simulink model "general_charger_2_with_new_rms"  (R2013a)
settings: Solver=ode45  StartTime=0  StopTime=2.5  RelTol=1e-3
PreLoadFcn:
  | Ts =5e-6;
values from neighbouring files (symbols this model uses):
  ac_volt = 169    [charger_init.m]    (also in charger_init_simpl.m)
  Cdc = 2e-3    (= 0.002)    [charger_init.m]    (also in charger_init_simpl.m)
  Lin = 1.5e-3    (= 0.0015)    [charger_init.m]    (also in charger_init_simpl.m = 0.001)
  P = 1.92e3    (= 1920)    [charger_init.m]    (also in charger_init_simpl.m)
  Q = 0    [charger_init.m]    (also in charger_init_simpl.m)
  ramp = (dc_volt - Vdcmin)/(acdc_ramp_end_time)    (= 202)    [charger_init.m]    (also in charger_init_simpl.m = (dc_volt - Vdcmin)/(acdc_ramp_end_time))
  switch_Ts = 5e-5    (= 5e-05)    [charger_init.m]    (also in charger_init_simpl.m)
  sys_Ts = 5e-6    (= 5e-06)    [charger_init.m]    (also in charger_init_simpl.m)
  Vdcmin = ac_volt + 10    (= 179)    [charger_init.m]    (also in charger_init_simpl.m)
  voc = 105    [charger_init.m]    (also in charger_init_simpl.m)
undefined symbols (not defined in the file or in its folder): CESR, DiscIntNeverNeededParam, Rin
undefined symbols (not defined in the file): active_power_on, Ad, Bd, Cd, dc_volt, dcdc_iki, dcdc_ikp, dcdc_on, dcdc_vki, dcdc_vkp, Dd, dq_id_ki, dq_id_kp, dq_iq_ki, dq_iq_kp, dq_vdc_ki, dq_vdc_kp, P_ki, P_kp, Q_ki, Q_kp, reactive_power_on
libraries: simulink_extras x132, powerlib x52, simulink x29, powerlib_meascontrol x8
(part 4 of 5)

== system general_charger_2_with_new_rms/Measurements/Power and angle calculations/discrete low pass filter1/Ad(1,3)/q rounder16 ==
  in : Inport
  Gain9 : Gain  Gain=2^-q
  Idealized ADC quantizer : simulink_extras/Additional Discrete/Idealized ADC quantizer  NumberOfConverterBits=32  Vmin=-range  Vmax=range  OutputDataType=double  OutputNegativeValues=on
  out : Outport
  wires:
  in/1 -> Idealized ADC quantizer/1
  Idealized ADC quantizer/1 -> Gain9/1
  Gain9/1 -> out/1

== system general_charger_2_with_new_rms/Measurements/Power and angle calculations/discrete low pass filter1/Ad(2,1)/q rounder16 ==
  in : Inport
  Gain9 : Gain  Gain=2^-q
  Idealized ADC quantizer : simulink_extras/Additional Discrete/Idealized ADC quantizer  NumberOfConverterBits=32  Vmin=-range  Vmax=range  OutputDataType=double  OutputNegativeValues=on
  out : Outport
  wires:
  in/1 -> Idealized ADC quantizer/1
  Idealized ADC quantizer/1 -> Gain9/1
  Gain9/1 -> out/1

== system general_charger_2_with_new_rms/Measurements/Power and angle calculations/discrete low pass filter1/Ad(2,2)/q rounder16 ==
  in : Inport
  Gain9 : Gain  Gain=2^-q
  Idealized ADC quantizer : simulink_extras/Additional Discrete/Idealized ADC quantizer  NumberOfConverterBits=32  Vmin=-range  Vmax=range  OutputDataType=double  OutputNegativeValues=on
  out : Outport
  wires:
  in/1 -> Idealized ADC quantizer/1
  Idealized ADC quantizer/1 -> Gain9/1
  Gain9/1 -> out/1

== system general_charger_2_with_new_rms/Measurements/Power and angle calculations/discrete low pass filter1/Ad(2,3)/q rounder16 ==
  in : Inport
  Gain9 : Gain  Gain=2^-q
  Idealized ADC quantizer : simulink_extras/Additional Discrete/Idealized ADC quantizer  NumberOfConverterBits=32  Vmin=-range  Vmax=range  OutputDataType=double  OutputNegativeValues=on
  out : Outport
  wires:
  in/1 -> Idealized ADC quantizer/1
  Idealized ADC quantizer/1 -> Gain9/1
  Gain9/1 -> out/1

== system general_charger_2_with_new_rms/Measurements/Power and angle calculations/discrete low pass filter1/Ad(3,1)/q rounder16 ==
  in : Inport
  Gain9 : Gain  Gain=2^-q
  Idealized ADC quantizer : simulink_extras/Additional Discrete/Idealized ADC quantizer  NumberOfConverterBits=32  Vmin=-range  Vmax=range  OutputDataType=double  OutputNegativeValues=on
  out : Outport
  wires:
  in/1 -> Idealized ADC quantizer/1
  Idealized ADC quantizer/1 -> Gain9/1
  Gain9/1 -> out/1

== system general_charger_2_with_new_rms/Measurements/Power and angle calculations/discrete low pass filter1/Ad(3,2)/q rounder16 ==
  in : Inport
  Gain9 : Gain  Gain=2^-q
  Idealized ADC quantizer : simulink_extras/Additional Discrete/Idealized ADC quantizer  NumberOfConverterBits=32  Vmin=-range  Vmax=range  OutputDataType=double  OutputNegativeValues=on
  out : Outport
  wires:
  in/1 -> Idealized ADC quantizer/1
  Idealized ADC quantizer/1 -> Gain9/1
  Gain9/1 -> out/1

== system general_charger_2_with_new_rms/Measurements/Power and angle calculations/discrete low pass filter1/Ad(3,3)/q rounder16 ==
  in : Inport
  Gain9 : Gain  Gain=2^-q
  Idealized ADC quantizer : simulink_extras/Additional Discrete/Idealized ADC quantizer  NumberOfConverterBits=32  Vmin=-range  Vmax=range  OutputDataType=double  OutputNegativeValues=on
  out : Outport
  wires:
  in/1 -> Idealized ADC quantizer/1
  Idealized ADC quantizer/1 -> Gain9/1
  Gain9/1 -> out/1

== system general_charger_2_with_new_rms/Measurements/Power and angle calculations/discrete low pass filter1/Bd(1)/q rounder16 ==
  in : Inport
  Gain9 : Gain  Gain=2^-q
  Idealized ADC quantizer : simulink_extras/Additional Discrete/Idealized ADC quantizer  NumberOfConverterBits=32  Vmin=-range  Vmax=range  OutputDataType=double  OutputNegativeValues=on
  out : Outport
  wires:
  in/1 -> Idealized ADC quantizer/1
  Idealized ADC quantizer/1 -> Gain9/1
  Gain9/1 -> out/1

== system general_charger_2_with_new_rms/Measurements/Power and angle calculations/discrete low pass filter1/Bd(2)/q rounder16 ==
  in : Inport
  Gain9 : Gain  Gain=2^-q
  Idealized ADC quantizer : simulink_extras/Additional Discrete/Idealized ADC quantizer  NumberOfConverterBits=32  Vmin=-range  Vmax=range  OutputDataType=double  OutputNegativeValues=on
  out : Outport
  wires:
  in/1 -> Idealized ADC quantizer/1
  Idealized ADC quantizer/1 -> Gain9/1
  Gain9/1 -> out/1

== system general_charger_2_with_new_rms/Measurements/Power and angle calculations/discrete low pass filter1/Bd(3)/q rounder16 ==
  in : Inport
  Gain9 : Gain  Gain=2^-q
  Idealized ADC quantizer : simulink_extras/Additional Discrete/Idealized ADC quantizer  NumberOfConverterBits=32  Vmin=-range  Vmax=range  OutputDataType=double  OutputNegativeValues=on
  out : Outport
  wires:
  in/1 -> Idealized ADC quantizer/1
  Idealized ADC quantizer/1 -> Gain9/1
  Gain9/1 -> out/1

== system general_charger_2_with_new_rms/Measurements/Power and angle calculations/discrete low pass filter1/Cd(1)/q rounder16 ==
  in : Inport
  Gain9 : Gain  Gain=2^-q
  Idealized ADC quantizer : simulink_extras/Additional Discrete/Idealized ADC quantizer  NumberOfConverterBits=32  Vmin=-range  Vmax=range  OutputDataType=double  OutputNegativeValues=on
  out : Outport
  wires:
  in/1 -> Idealized ADC quantizer/1
  Idealized ADC quantizer/1 -> Gain9/1
  Gain9/1 -> out/1

== system general_charger_2_with_new_rms/Measurements/Power and angle calculations/discrete low pass filter1/Cd(2)/q rounder16 ==
  in : Inport
  Gain9 : Gain  Gain=2^-q
  Idealized ADC quantizer : simulink_extras/Additional Discrete/Idealized ADC quantizer  NumberOfConverterBits=32  Vmin=-range  Vmax=range  OutputDataType=double  OutputNegativeValues=on
  out : Outport
  wires:
  in/1 -> Idealized ADC quantizer/1
  Idealized ADC quantizer/1 -> Gain9/1
  Gain9/1 -> out/1

== system general_charger_2_with_new_rms/Measurements/Power and angle calculations/discrete low pass filter1/Cd(3)/q rounder16 ==
  in : Inport
  Gain9 : Gain  Gain=2^-q
  Idealized ADC quantizer : simulink_extras/Additional Discrete/Idealized ADC quantizer  NumberOfConverterBits=32  Vmin=-range  Vmax=range  OutputDataType=double  OutputNegativeValues=on
  out : Outport
  wires:
  in/1 -> Idealized ADC quantizer/1
  Idealized ADC quantizer/1 -> Gain9/1
  Gain9/1 -> out/1

== system general_charger_2_with_new_rms/Measurements/Power and angle calculations/discrete low pass filter1/Dd/q rounder16 ==
  in : Inport
  Gain9 : Gain  Gain=2^-q
  Idealized ADC quantizer : simulink_extras/Additional Discrete/Idealized ADC quantizer  NumberOfConverterBits=32  Vmin=-range  Vmax=range  OutputDataType=double  OutputNegativeValues=on
  out : Outport
  wires:
  in/1 -> Idealized ADC quantizer/1
  Idealized ADC quantizer/1 -> Gain9/1
  Gain9/1 -> out/1

== system general_charger_2_with_new_rms/Measurements/Power and angle calculations/discrete low pass filter2/Ad(1,1)/q rounder16 ==
  in : Inport
  Gain9 : Gain  Gain=2^-q
  Idealized ADC quantizer : simulink_extras/Additional Discrete/Idealized ADC quantizer  NumberOfConverterBits=32  Vmin=-range  Vmax=range  OutputDataType=double  OutputNegativeValues=on
  out : Outport
  wires:
  in/1 -> Idealized ADC quantizer/1
  Idealized ADC quantizer/1 -> Gain9/1
  Gain9/1 -> out/1

== system general_charger_2_with_new_rms/Measurements/Power and angle calculations/discrete low pass filter2/Ad(1,2)/q rounder16 ==
  in : Inport
  Gain9 : Gain  Gain=2^-q
  Idealized ADC quantizer : simulink_extras/Additional Discrete/Idealized ADC quantizer  NumberOfConverterBits=32  Vmin=-range  Vmax=range  OutputDataType=double  OutputNegativeValues=on
  out : Outport
  wires:
  in/1 -> Idealized ADC quantizer/1
  Idealized ADC quantizer/1 -> Gain9/1
  Gain9/1 -> out/1

== system general_charger_2_with_new_rms/Measurements/Power and angle calculations/discrete low pass filter2/Ad(1,3)/q rounder16 ==
  in : Inport
  Gain9 : Gain  Gain=2^-q
  Idealized ADC quantizer : simulink_extras/Additional Discrete/Idealized ADC quantizer  NumberOfConverterBits=32  Vmin=-range  Vmax=range  OutputDataType=double  OutputNegativeValues=on
  out : Outport
  wires:
  in/1 -> Idealized ADC quantizer/1
  Idealized ADC quantizer/1 -> Gain9/1
  Gain9/1 -> out/1

== system general_charger_2_with_new_rms/Measurements/Power and angle calculations/discrete low pass filter2/Ad(2,1)/q rounder16 ==
  in : Inport
  Gain9 : Gain  Gain=2^-q
  Idealized ADC quantizer : simulink_extras/Additional Discrete/Idealized ADC quantizer  NumberOfConverterBits=32  Vmin=-range  Vmax=range  OutputDataType=double  OutputNegativeValues=on
  out : Outport
  wires:
  in/1 -> Idealized ADC quantizer/1
  Idealized ADC quantizer/1 -> Gain9/1
  Gain9/1 -> out/1

== system general_charger_2_with_new_rms/Measurements/Power and angle calculations/discrete low pass filter2/Ad(2,2)/q rounder16 ==
  in : Inport
  Gain9 : Gain  Gain=2^-q
  Idealized ADC quantizer : simulink_extras/Additional Discrete/Idealized ADC quantizer  NumberOfConverterBits=32  Vmin=-range  Vmax=range  OutputDataType=double  OutputNegativeValues=on
  out : Outport
  wires:
  in/1 -> Idealized ADC quantizer/1
  Idealized ADC quantizer/1 -> Gain9/1
  Gain9/1 -> out/1

== system general_charger_2_with_new_rms/Measurements/Power and angle calculations/discrete low pass filter2/Ad(2,3)/q rounder16 ==
  in : Inport
  Gain9 : Gain  Gain=2^-q
  Idealized ADC quantizer : simulink_extras/Additional Discrete/Idealized ADC quantizer  NumberOfConverterBits=32  Vmin=-range  Vmax=range  OutputDataType=double  OutputNegativeValues=on
  out : Outport
  wires:
  in/1 -> Idealized ADC quantizer/1
  Idealized ADC quantizer/1 -> Gain9/1
  Gain9/1 -> out/1

== system general_charger_2_with_new_rms/Measurements/Power and angle calculations/discrete low pass filter2/Ad(3,1)/q rounder16 ==
  in : Inport
  Gain9 : Gain  Gain=2^-q
  Idealized ADC quantizer : simulink_extras/Additional Discrete/Idealized ADC quantizer  NumberOfConverterBits=32  Vmin=-range  Vmax=range  OutputDataType=double  OutputNegativeValues=on
  out : Outport
  wires:
  in/1 -> Idealized ADC quantizer/1
  Idealized ADC quantizer/1 -> Gain9/1
  Gain9/1 -> out/1

== system general_charger_2_with_new_rms/Measurements/Power and angle calculations/discrete low pass filter2/Ad(3,2)/q rounder16 ==
  in : Inport
  Gain9 : Gain  Gain=2^-q
  Idealized ADC quantizer : simulink_extras/Additional Discrete/Idealized ADC quantizer  NumberOfConverterBits=32  Vmin=-range  Vmax=range  OutputDataType=double  OutputNegativeValues=on
  out : Outport
  wires:
  in/1 -> Idealized ADC quantizer/1
  Idealized ADC quantizer/1 -> Gain9/1
  Gain9/1 -> out/1

== system general_charger_2_with_new_rms/Measurements/Power and angle calculations/discrete low pass filter2/Ad(3,3)/q rounder16 ==
  in : Inport
  Gain9 : Gain  Gain=2^-q
  Idealized ADC quantizer : simulink_extras/Additional Discrete/Idealized ADC quantizer  NumberOfConverterBits=32  Vmin=-range  Vmax=range  OutputDataType=double  OutputNegativeValues=on
  out : Outport
  wires:
  in/1 -> Idealized ADC quantizer/1
  Idealized ADC quantizer/1 -> Gain9/1
  Gain9/1 -> out/1

== system general_charger_2_with_new_rms/Measurements/Power and angle calculations/discrete low pass filter2/Bd(1)/q rounder16 ==
  in : Inport
  Gain9 : Gain  Gain=2^-q
  Idealized ADC quantizer : simulink_extras/Additional Discrete/Idealized ADC quantizer  NumberOfConverterBits=32  Vmin=-range  Vmax=range  OutputDataType=double  OutputNegativeValues=on
  out : Outport
  wires:
  in/1 -> Idealized ADC quantizer/1
  Idealized ADC quantizer/1 -> Gain9/1
  Gain9/1 -> out/1

== system general_charger_2_with_new_rms/Measurements/Power and angle calculations/discrete low pass filter2/Bd(2)/q rounder16 ==
  in : Inport
  Gain9 : Gain  Gain=2^-q
  Idealized ADC quantizer : simulink_extras/Additional Discrete/Idealized ADC quantizer  NumberOfConverterBits=32  Vmin=-range  Vmax=range  OutputDataType=double  OutputNegativeValues=on
  out : Outport
  wires:
  in/1 -> Idealized ADC quantizer/1
  Idealized ADC quantizer/1 -> Gain9/1
  Gain9/1 -> out/1

== system general_charger_2_with_new_rms/Measurements/Power and angle calculations/discrete low pass filter2/Bd(3)/q rounder16 ==
  in : Inport
  Gain9 : Gain  Gain=2^-q
  Idealized ADC quantizer : simulink_extras/Additional Discrete/Idealized ADC quantizer  NumberOfConverterBits=32  Vmin=-range  Vmax=range  OutputDataType=double  OutputNegativeValues=on
  out : Outport
  wires:
  in/1 -> Idealized ADC quantizer/1
  Idealized ADC quantizer/1 -> Gain9/1
  Gain9/1 -> out/1

== system general_charger_2_with_new_rms/Measurements/Power and angle calculations/discrete low pass filter2/Cd(1)/q rounder16 ==
  in : Inport
  Gain9 : Gain  Gain=2^-q
  Idealized ADC quantizer : simulink_extras/Additional Discrete/Idealized ADC quantizer  NumberOfConverterBits=32  Vmin=-range  Vmax=range  OutputDataType=double  OutputNegativeValues=on
  out : Outport
  wires:
  in/1 -> Idealized ADC quantizer/1
  Idealized ADC quantizer/1 -> Gain9/1
  Gain9/1 -> out/1

== system general_charger_2_with_new_rms/Measurements/Power and angle calculations/discrete low pass filter2/Cd(2)/q rounder16 ==
  in : Inport
  Gain9 : Gain  Gain=2^-q
  Idealized ADC quantizer : simulink_extras/Additional Discrete/Idealized ADC quantizer  NumberOfConverterBits=32  Vmin=-range  Vmax=range  OutputDataType=double  OutputNegativeValues=on
  out : Outport
  wires:
  in/1 -> Idealized ADC quantizer/1
  Idealized ADC quantizer/1 -> Gain9/1
  Gain9/1 -> out/1

== system general_charger_2_with_new_rms/Measurements/Power and angle calculations/discrete low pass filter2/Cd(3)/q rounder16 ==
  in : Inport
  Gain9 : Gain  Gain=2^-q
  Idealized ADC quantizer : simulink_extras/Additional Discrete/Idealized ADC quantizer  NumberOfConverterBits=32  Vmin=-range  Vmax=range  OutputDataType=double  OutputNegativeValues=on
  out : Outport
  wires:
  in/1 -> Idealized ADC quantizer/1
  Idealized ADC quantizer/1 -> Gain9/1
  Gain9/1 -> out/1

== system general_charger_2_with_new_rms/Measurements/Power and angle calculations/discrete low pass filter2/Dd/q rounder16 ==
  in : Inport
  Gain9 : Gain  Gain=2^-q
  Idealized ADC quantizer : simulink_extras/Additional Discrete/Idealized ADC quantizer  NumberOfConverterBits=32  Vmin=-range  Vmax=range  OutputDataType=double  OutputNegativeValues=on
  out : Outport
  wires:
  in/1 -> Idealized ADC quantizer/1
  Idealized ADC quantizer/1 -> Gain9/1
  Gain9/1 -> out/1

== system general_charger_2_with_new_rms/Measurements/THD/discrete low pass filter1/Ad(1,1)/q rounder16 ==
  in : Inport
  Gain9 : Gain  Gain=2^-q
  Idealized ADC quantizer : simulink_extras/Additional Discrete/Idealized ADC quantizer  NumberOfConverterBits=32  Vmin=-range  Vmax=range  OutputDataType=double  OutputNegativeValues=on
  out : Outport
  wires:
  in/1 -> Idealized ADC quantizer/1
  Idealized ADC quantizer/1 -> Gain9/1
  Gain9/1 -> out/1

== system general_charger_2_with_new_rms/Measurements/THD/discrete low pass filter1/Ad(1,2)/q rounder16 ==
  in : Inport
  Gain9 : Gain  Gain=2^-q
  Idealized ADC quantizer : simulink_extras/Additional Discrete/Idealized ADC quantizer  NumberOfConverterBits=32  Vmin=-range  Vmax=range  OutputDataType=double  OutputNegativeValues=on
  out : Outport
  wires:
  in/1 -> Idealized ADC quantizer/1
  Idealized ADC quantizer/1 -> Gain9/1
  Gain9/1 -> out/1

== system general_charger_2_with_new_rms/Measurements/THD/discrete low pass filter1/Ad(1,3)/q rounder16 ==
  in : Inport
  Gain9 : Gain  Gain=2^-q
  Idealized ADC quantizer : simulink_extras/Additional Discrete/Idealized ADC quantizer  NumberOfConverterBits=32  Vmin=-range  Vmax=range  OutputDataType=double  OutputNegativeValues=on
  out : Outport
  wires:
  in/1 -> Idealized ADC quantizer/1
  Idealized ADC quantizer/1 -> Gain9/1
  Gain9/1 -> out/1

== system general_charger_2_with_new_rms/Measurements/THD/discrete low pass filter1/Ad(2,1)/q rounder16 ==
  in : Inport
  Gain9 : Gain  Gain=2^-q
  Idealized ADC quantizer : simulink_extras/Additional Discrete/Idealized ADC quantizer  NumberOfConverterBits=32  Vmin=-range  Vmax=range  OutputDataType=double  OutputNegativeValues=on
  out : Outport
  wires:
  in/1 -> Idealized ADC quantizer/1
  Idealized ADC quantizer/1 -> Gain9/1
  Gain9/1 -> out/1

== system general_charger_2_with_new_rms/Measurements/THD/discrete low pass filter1/Ad(2,2)/q rounder16 ==
  in : Inport
  Gain9 : Gain  Gain=2^-q
  Idealized ADC quantizer : simulink_extras/Additional Discrete/Idealized ADC quantizer  NumberOfConverterBits=32  Vmin=-range  Vmax=range  OutputDataType=double  OutputNegativeValues=on
  out : Outport
  wires:
  in/1 -> Idealized ADC quantizer/1
  Idealized ADC quantizer/1 -> Gain9/1
  Gain9/1 -> out/1

== system general_charger_2_with_new_rms/Measurements/THD/discrete low pass filter1/Ad(2,3)/q rounder16 ==
  in : Inport
  Gain9 : Gain  Gain=2^-q
  Idealized ADC quantizer : simulink_extras/Additional Discrete/Idealized ADC quantizer  NumberOfConverterBits=32  Vmin=-range  Vmax=range  OutputDataType=double  OutputNegativeValues=on
  out : Outport
  wires:
  in/1 -> Idealized ADC quantizer/1
  Idealized ADC quantizer/1 -> Gain9/1
  Gain9/1 -> out/1

== system general_charger_2_with_new_rms/Measurements/THD/discrete low pass filter1/Ad(3,1)/q rounder16 ==
  in : Inport
  Gain9 : Gain  Gain=2^-q
  Idealized ADC quantizer : simulink_extras/Additional Discrete/Idealized ADC quantizer  NumberOfConverterBits=32  Vmin=-range  Vmax=range  OutputDataType=double  OutputNegativeValues=on
  out : Outport
  wires:
  in/1 -> Idealized ADC quantizer/1
  Idealized ADC quantizer/1 -> Gain9/1
  Gain9/1 -> out/1

== system general_charger_2_with_new_rms/Measurements/THD/discrete low pass filter1/Ad(3,2)/q rounder16 ==
  in : Inport
  Gain9 : Gain  Gain=2^-q
  Idealized ADC quantizer : simulink_extras/Additional Discrete/Idealized ADC quantizer  NumberOfConverterBits=32  Vmin=-range  Vmax=range  OutputDataType=double  OutputNegativeValues=on
  out : Outport
  wires:
  in/1 -> Idealized ADC quantizer/1
  Idealized ADC quantizer/1 -> Gain9/1
  Gain9/1 -> out/1

== system general_charger_2_with_new_rms/Measurements/THD/discrete low pass filter1/Ad(3,3)/q rounder16 ==
  in : Inport
  Gain9 : Gain  Gain=2^-q
  Idealized ADC quantizer : simulink_extras/Additional Discrete/Idealized ADC quantizer  NumberOfConverterBits=32  Vmin=-range  Vmax=range  OutputDataType=double  OutputNegativeValues=on
  out : Outport
  wires:
  in/1 -> Idealized ADC quantizer/1
  Idealized ADC quantizer/1 -> Gain9/1
  Gain9/1 -> out/1

== system general_charger_2_with_new_rms/Measurements/THD/discrete low pass filter1/Bd(1)/q rounder16 ==
  in : Inport
  Gain9 : Gain  Gain=2^-q
  Idealized ADC quantizer : simulink_extras/Additional Discrete/Idealized ADC quantizer  NumberOfConverterBits=32  Vmin=-range  Vmax=range  OutputDataType=double  OutputNegativeValues=on
  out : Outport
  wires:
  in/1 -> Idealized ADC quantizer/1
  Idealized ADC quantizer/1 -> Gain9/1
  Gain9/1 -> out/1

== system general_charger_2_with_new_rms/Measurements/THD/discrete low pass filter1/Bd(2)/q rounder16 ==
  in : Inport
  Gain9 : Gain  Gain=2^-q
  Idealized ADC quantizer : simulink_extras/Additional Discrete/Idealized ADC quantizer  NumberOfConverterBits=32  Vmin=-range  Vmax=range  OutputDataType=double  OutputNegativeValues=on
  out : Outport
  wires:
  in/1 -> Idealized ADC quantizer/1
  Idealized ADC quantizer/1 -> Gain9/1
  Gain9/1 -> out/1

== system general_charger_2_with_new_rms/Measurements/THD/discrete low pass filter1/Bd(3)/q rounder16 ==
  in : Inport
  Gain9 : Gain  Gain=2^-q
  Idealized ADC quantizer : simulink_extras/Additional Discrete/Idealized ADC quantizer  NumberOfConverterBits=32  Vmin=-range  Vmax=range  OutputDataType=double  OutputNegativeValues=on
  out : Outport
  wires:
  in/1 -> Idealized ADC quantizer/1
  Idealized ADC quantizer/1 -> Gain9/1
  Gain9/1 -> out/1

== system general_charger_2_with_new_rms/Measurements/THD/discrete low pass filter1/Cd(1)/q rounder16 ==
  in : Inport
  Gain9 : Gain  Gain=2^-q
  Idealized ADC quantizer : simulink_extras/Additional Discrete/Idealized ADC quantizer  NumberOfConverterBits=32  Vmin=-range  Vmax=range  OutputDataType=double  OutputNegativeValues=on
  out : Outport
  wires:
  in/1 -> Idealized ADC quantizer/1
  Idealized ADC quantizer/1 -> Gain9/1
  Gain9/1 -> out/1

== system general_charger_2_with_new_rms/Measurements/THD/discrete low pass filter1/Cd(2)/q rounder16 ==
  in : Inport
  Gain9 : Gain  Gain=2^-q
  Idealized ADC quantizer : simulink_extras/Additional Discrete/Idealized ADC quantizer  NumberOfConverterBits=32  Vmin=-range  Vmax=range  OutputDataType=double  OutputNegativeValues=on
  out : Outport
  wires:
  in/1 -> Idealized ADC quantizer/1
  Idealized ADC quantizer/1 -> Gain9/1
  Gain9/1 -> out/1

== system general_charger_2_with_new_rms/Measurements/THD/discrete low pass filter1/Cd(3)/q rounder16 ==
  in : Inport
  Gain9 : Gain  Gain=2^-q
  Idealized ADC quantizer : simulink_extras/Additional Discrete/Idealized ADC quantizer  NumberOfConverterBits=32  Vmin=-range  Vmax=range  OutputDataType=double  OutputNegativeValues=on
  out : Outport
  wires:
  in/1 -> Idealized ADC quantizer/1
  Idealized ADC quantizer/1 -> Gain9/1
  Gain9/1 -> out/1

== system general_charger_2_with_new_rms/Measurements/THD/discrete low pass filter1/Dd/q rounder16 ==
  in : Inport
  Gain9 : Gain  Gain=2^-q
  Idealized ADC quantizer : simulink_extras/Additional Discrete/Idealized ADC quantizer  NumberOfConverterBits=32  Vmin=-range  Vmax=range  OutputDataType=double  OutputNegativeValues=on
  out : Outport
  wires:
  in/1 -> Idealized ADC quantizer/1
  Idealized ADC quantizer/1 -> Gain9/1
  Gain9/1 -> out/1

== system general_charger_2_with_new_rms/control_stage/AC//DC Control/DQ Controller/AB-DQ Transform/AB->DQ ==
  A : Inport
  wt : Inport  Port=2
  phi : Inport  Port=3
  Add1 : Sum  Inputs=-+
  Add2 : Sum
  Delay : Delay  DelayLength=RSpC  SampleTime=abdq_Ts
  Gain : Gain  Gain=-1
  Id Discretization Error Correction : Subsystem
  Iq Discretization Error Correction : Subsystem
  Product{1..4} (4 alike) : Product  RndMeth=Zero
  Trigonometric Function : Trigonometry
  Trigonometric Function1 : Trigonometry  Operator=cos
  Unit Delay : UnitDelay  SampleTime=switch_Ts
  D : Outport
  Q : Outport  Port=2
  wires:
  Trigonometric Function/1 -> Product1/1, Product2/1
  Product1/1 -> Add2/2
  Product4/1 -> Add2/1
  Product2/1 -> Add1/1
  A/1 -> Iq Discretization Error Correction/4(A), Delay/1, Id Discretization Error Correction/1(A), Product4/1, Product2/2
  Trigonometric Function1/1 -> Product4/2, Product3/1
  Product3/1 -> Add1/2
  Delay/1 -> Product1/2, Product3/2  "B"
  wt/1 -> [theta], Trigonometric Function1/1, Trigonometric Function/1
  Add2/1 -> Id Discretization Error Correction/3(D)  "Vd"
  Add1/1 -> Iq Discretization Error Correction/2(Q)
  [theta] -> Iq Discretization Error Correction/3(wt)
  [theta] -> Id Discretization Error Correction/2(wt)
  Id Discretization Error Correction/1(Id_corr) -> D/1
  Iq Discretization Error Correction/1(Iq_corr) -> Q/1
  phi/1 -> Gain/1
  Unit Delay/1 -> Iq Discretization Error Correction/1(phi), Id Discretization Error Correction/4(phi)
  Gain/1 -> Unit Delay/1

== system general_charger_2_with_new_rms/control_stage/AC//DC Control/DQ Controller/AB-DQ Transform/PLL ==
  note: PLL based on dq frame control
      | input signal is assumed to be 60 Hz
      | and sample time is 50e-6
  signal_in : Inport
  AB->DQ : Subsystem  mask{abdq_f=pll_f, abdq_Ts=pll_Ts}
      mask prompts: abdq_f "frequency"; abdq_Ts "Sample Time"
      mask init:
      | SpC=1/abdq_f/4/abdq_Ts;
      | RSpC=ceil(SpC);
  Constant1 : Constant  Value=0
  Constant3 : Constant  Value=2*pi*pll_f
  PI1 : Subsystem  mask{ki=1, kp=0, Ts_pi=pll_Ts, int_sat_up=inf, int_sat_low=-inf, pi_sat_up=inf, pi_sat_low=-inf}
      mask prompts: ki "Integral Gain"; kp "Proportional Gain"; Ts_pi "Sample Time"; int_sat_up "Integral Saturation Upper"; int_sat_low "Integral Saturation Lower"; pi_sat_up "PI Controller Saturation Upper"; pi_sat_low "PI Controller Saturation Lower"
      mask Display: disp('PI')
  PI4 : Subsystem  mask{ki=pll_ki, kp=pll_kp, Ts_pi=pll_Ts, int_sat_up=inf, int_sat_low=-inf, pi_sat_up=inf, pi_sat_low=-inf}
      mask prompts: ki "Integral Gain"; kp "Proportional Gain"; Ts_pi "Sample Time"; int_sat_up "Integral Saturation Upper"; int_sat_low "Integral Saturation Lower"; pi_sat_up "PI Controller Saturation Upper"; pi_sat_low "PI Controller Saturation Lower"
      mask Display: disp('PI')
  Sum : Sum  Inputs=|-+
  Sum2 : Sum  Inputs=|-+
  angle_out : Outport
  D : Outport  Port=2
  Q : Outport  Port=3
  wires:
  Constant1/1 -> Sum/2
  Sum/1 -> PI4/1(in)
  PI1/1(out) -> angle_out/1, AB->DQ/2(wt)
  Constant3/1 -> Sum2/2
  PI4/1(out) -> Sum2/1
  AB->DQ/2(Q) -> Q/1, Sum/1
  signal_in/1 -> AB->DQ/1(A)
  AB->DQ/1(D) -> D/1
  Sum2/1 -> PI1/1(in)  "pll_int_error"

== system general_charger_2_with_new_rms/control_stage/AC//DC Control/DQ Controller/DQ Controller Submodule/DQ-->A ==
  D : Inport
  Q : Inport  Port=2
  wt : Inport  Port=3
  Add2 : Sum  Inputs=+-
  Product1 : Product  RndMeth=Zero
  Product4 : Product  RndMeth=Zero
  Trigonometric Function : Trigonometry
  Trigonometric Function1 : Trigonometry  Operator=cos
  A : Outport
  wires:
  Add2/1 -> A/1  "Vd"
  Product1/1 -> Add2/2
  Product4/1 -> Add2/1
  wt/1 -> Trigonometric Function1/1, Trigonometric Function/1
  Trigonometric Function1/1 -> Product4/2
  D/1 -> Product4/1
  Q/1 -> Product1/2
  Trigonometric Function/1 -> Product1/1

== system general_charger_2_with_new_rms/control_stage/AC//DC Control/DQ Controller/DQ Controller Submodule/PI1 ==
  in : Inport
  Add1 : Sum
  Add2 : Sum
  Ki : Gain  Gain=ki
  Kp : Gain  Gain=kp
  Tappe : simulink/Discrete/Tapped Delay  vinit=0.0  samptime=Ts_pi  NumDelays=1  DelayOrder=Oldest  includeCurrent=off
  Ts : Gain  Gain=Ts_pi
  integral saturation : Saturate  UpperLimit=int_sat_up  LowerLimit=int_sat_low  SampleTime=Ts_pi
  pi controller saturation : Saturate  UpperLimit=pi_sat_up  LowerLimit=pi_sat_low  SampleTime=Ts_pi
  out : Outport
  wires:
  Ts/1 -> Ki/1
  in/1 -> Kp/1, Ts/1  "vdc_error"
  Add1/1 -> integral saturation/1  "vdc_int_pi"
  Kp/1 -> Add2/2  "vdc_kp_pi"
  pi controller saturation/1 -> out/1
  Tappe/1 -> Add1/1
  Add2/1 -> pi controller saturation/1  "vdc_pi"
  Ki/1 -> Add1/2
  integral saturation/1 -> Add2/1, Tappe/1

== system general_charger_2_with_new_rms/control_stage/AC//DC Control/DQ Controller/DQ Controller Submodule/PI2 ==
  in : Inport
  Add1 : Sum
  Add2 : Sum
  Ki : Gain  Gain=ki
  Kp : Gain  Gain=kp
  Tappe : simulink/Discrete/Tapped Delay  vinit=0.0  samptime=Ts_pi  NumDelays=1  DelayOrder=Oldest  includeCurrent=off
  Ts : Gain  Gain=Ts_pi
  integral saturation : Saturate  UpperLimit=int_sat_up  LowerLimit=int_sat_low  SampleTime=Ts_pi
  pi controller saturation : Saturate  UpperLimit=pi_sat_up  LowerLimit=pi_sat_low  SampleTime=Ts_pi
  out : Outport
  wires:
  Ts/1 -> Ki/1
  in/1 -> Kp/1, Ts/1  "vdc_error"
  Add1/1 -> integral saturation/1  "vdc_int_pi"
  Kp/1 -> Add2/2  "vdc_kp_pi"
  pi controller saturation/1 -> out/1
  Tappe/1 -> Add1/1
  Add2/1 -> pi controller saturation/1  "vdc_pi"
  Ki/1 -> Add1/2
  integral saturation/1 -> Add2/1, Tappe/1

== system general_charger_2_with_new_rms/control_stage/AC//DC Control/DQ Controller/DQ Controller Submodule/PI3 ==
  in : Inport
  Add1 : Sum
  Add2 : Sum
  Ki : Gain  Gain=ki
  Kp : Gain  Gain=kp
  Tappe : simulink/Discrete/Tapped Delay  vinit=0.0  samptime=Ts_pi  NumDelays=1  DelayOrder=Oldest  includeCurrent=off
  Ts : Gain  Gain=Ts_pi
  integral saturation : Saturate  UpperLimit=int_sat_up  LowerLimit=int_sat_low  SampleTime=Ts_pi
  pi controller saturation : Saturate  UpperLimit=pi_sat_up  LowerLimit=pi_sat_low  SampleTime=Ts_pi
  out : Outport
  wires:
  Ts/1 -> Ki/1
  in/1 -> Kp/1, Ts/1  "vdc_error"
  Add1/1 -> integral saturation/1  "vdc_int_pi"
  Kp/1 -> Add2/2  "vdc_kp_pi"
  pi controller saturation/1 -> out/1
  Tappe/1 -> Add1/1
  Add2/1 -> pi controller saturation/1  "vdc_pi"
  Ki/1 -> Add1/2
  integral saturation/1 -> Add2/1, Tappe/1

== system general_charger_2_with_new_rms/control_stage/AC//DC Control/DQ Controller/DQ Controller Submodule/Reactive Power Control Module ==
  Add8 : Sum  Inputs=+-
  Constant1 : Constant  Value=Q
  Constant3 : Constant  Value=0
  Divide2 : Product  Inputs=/*  InputSameDT=on
  Gain4 : Gain  Gain=0.5
  Gain5 : Gain  Gain=-1
  PI4 : Subsystem  mask{ki=Q_ki, kp=Q_kp, Ts_pi=Ts, int_sat_up=inf, int_sat_low=-inf, pi_sat_up=inf, pi_sat_low=-inf}
      mask prompts: ki "Integral Gain"; kp "Proportional Gain"; Ts_pi "Sample Time"; int_sat_up "Integral Saturation Upper"; int_sat_low "Integral Saturation Lower"; pi_sat_up "PI Controller Saturation Upper"; pi_sat_low "PI Controller Saturation Lower"
      mask Display: disp('PI')
  Saturation : Saturate  UpperLimit=inf  LowerLimit=1
  Step1 : Step  Time=turn_on  SampleTime=0
  Switch3 : Switch  Threshold=0.5
  Iq_ref : Outport
  wires:
  PI4/1(out) -> Iq_ref/1
  Gain4/1 -> Divide2/1
  Divide2/1 -> PI4/1(in)
  Saturation/1 -> Gain4/1
  Gain5/1 -> Switch3/1
  Constant3/1 -> Switch3/3
  Constant1/1 -> Add8/1
  [Qpower] -> Add8/2
  Step1/1 -> Switch3/2
  [nVd] -> Saturation/1
  Switch3/1 -> Divide2/2
  Add8/1 -> Gain5/1

== system general_charger_2_with_new_rms/control_stage/AC//DC Control/DQ Controller/discrete low pass filter1/Ad(1,1) ==
  in : Inport
  Constant1 : Constant  Value=variable
  Product1 : Product
  q rounder16 : Subsystem  mask{q=nQ, range=maxRange}
      mask prompts: q "q value"; range "q range"
  out : Outport
  wires:
  q rounder16/1(out) -> Product1/1
  Constant1/1 -> q rounder16/1(in)
  Product1/1 -> out/1
  in/1 -> Product1/2

== system general_charger_2_with_new_rms/control_stage/AC//DC Control/DQ Controller/discrete low pass filter1/Ad(1,2) ==
  in : Inport
  Constant1 : Constant  Value=variable
  Product1 : Product
  q rounder16 : Subsystem  mask{q=nQ, range=maxRange}
      mask prompts: q "q value"; range "q range"
  out : Outport
  wires:
  q rounder16/1(out) -> Product1/1
  Constant1/1 -> q rounder16/1(in)
  Product1/1 -> out/1
  in/1 -> Product1/2

== system general_charger_2_with_new_rms/control_stage/AC//DC Control/DQ Controller/discrete low pass filter1/Ad(1,3) ==
  in : Inport
  Constant1 : Constant  Value=variable
  Product1 : Product
  Scope1 : Scope  NumInputPorts=2
      settings: YMin=-5~-5  YMax=5~5
  q rounder16 : Subsystem  mask{q=nQ, range=maxRange}
      mask prompts: q "q value"; range "q range"
  out : Outport
  wires:
  q rounder16/1(out) -> Product1/1, Scope1/2
  Constant1/1 -> Scope1/1, q rounder16/1(in)
  Product1/1 -> out/1
  in/1 -> Product1/2

== system general_charger_2_with_new_rms/control_stage/AC//DC Control/DQ Controller/discrete low pass filter1/Ad(2,1) ==
  in : Inport
  Constant1 : Constant  Value=variable
  Product1 : Product
  Scope1 : Scope  NumInputPorts=2
      settings: YMin=-5~-5  YMax=5~5
  q rounder16 : Subsystem  mask{q=nQ, range=maxRange}
      mask prompts: q "q value"; range "q range"
  out : Outport
  wires:
  q rounder16/1(out) -> Product1/1, Scope1/2
  Constant1/1 -> Scope1/1, q rounder16/1(in)
  Product1/1 -> out/1
  in/1 -> Product1/2

== system general_charger_2_with_new_rms/control_stage/AC//DC Control/DQ Controller/discrete low pass filter1/Ad(2,2) ==
  in : Inport
  Constant1 : Constant  Value=variable
  Product1 : Product
  Scope1 : Scope  NumInputPorts=2
      settings: YMin=-5~-5  YMax=5~5
  q rounder16 : Subsystem  mask{q=nQ, range=maxRange}
      mask prompts: q "q value"; range "q range"
  out : Outport
  wires:
  q rounder16/1(out) -> Product1/1, Scope1/2
  Constant1/1 -> Scope1/1, q rounder16/1(in)
  Product1/1 -> out/1
  in/1 -> Product1/2

== system general_charger_2_with_new_rms/control_stage/AC//DC Control/DQ Controller/discrete low pass filter1/Ad(2,3) ==
  in : Inport
  Constant1 : Constant  Value=variable
  Product1 : Product
  Scope1 : Scope  NumInputPorts=2
      settings: YMin=-5~-5  YMax=5~5
  q rounder16 : Subsystem  mask{q=nQ, range=maxRange}
      mask prompts: q "q value"; range "q range"
  out : Outport
  wires:
  q rounder16/1(out) -> Product1/1, Scope1/2
  Constant1/1 -> Scope1/1, q rounder16/1(in)
  Product1/1 -> out/1
  in/1 -> Product1/2

== system general_charger_2_with_new_rms/control_stage/AC//DC Control/DQ Controller/discrete low pass filter1/Ad(3,1) ==
  in : Inport
  Constant1 : Constant  Value=variable
  Product1 : Product
  Scope1 : Scope  NumInputPorts=2
      settings: YMin=-5~-5  YMax=5~5
  q rounder16 : Subsystem  mask{q=nQ, range=maxRange}
      mask prompts: q "q value"; range "q range"
  out : Outport
  wires:
  q rounder16/1(out) -> Product1/1, Scope1/2
  Constant1/1 -> Scope1/1, q rounder16/1(in)
  Product1/1 -> out/1
  in/1 -> Product1/2

== system general_charger_2_with_new_rms/control_stage/AC//DC Control/DQ Controller/discrete low pass filter1/Ad(3,2) ==
  in : Inport
  Constant1 : Constant  Value=variable
  Product1 : Product
  Scope1 : Scope  NumInputPorts=2
      settings: YMin=-5~-5  YMax=5~5
  q rounder16 : Subsystem  mask{q=nQ, range=maxRange}
      mask prompts: q "q value"; range "q range"
  out : Outport
  wires:
  q rounder16/1(out) -> Product1/1, Scope1/2
  Constant1/1 -> Scope1/1, q rounder16/1(in)
  Product1/1 -> out/1
  in/1 -> Product1/2

== system general_charger_2_with_new_rms/control_stage/AC//DC Control/DQ Controller/discrete low pass filter1/Ad(3,3) ==
  in : Inport
  Constant1 : Constant  Value=variable
  Product1 : Product
  Scope1 : Scope  NumInputPorts=2
      settings: YMin=-5~-5  YMax=5~5
  q rounder16 : Subsystem  mask{q=nQ, range=maxRange}
      mask prompts: q "q value"; range "q range"
  out : Outport
  wires:
  q rounder16/1(out) -> Product1/1, Scope1/2
  Constant1/1 -> Scope1/1, q rounder16/1(in)
  Product1/1 -> out/1
  in/1 -> Product1/2

== system general_charger_2_with_new_rms/control_stage/AC//DC Control/DQ Controller/discrete low pass filter1/Bd(1) ==
  in : Inport
  Constant1 : Constant  Value=variable
  Product1 : Product
  q rounder16 : Subsystem  mask{q=nQ, range=maxRange}
      mask prompts: q "q value"; range "q range"
  out : Outport
  wires:
  q rounder16/1(out) -> Product1/1
  Constant1/1 -> q rounder16/1(in)
  Product1/1 -> out/1
  in/1 -> Product1/2

== system general_charger_2_with_new_rms/control_stage/AC//DC Control/DQ Controller/discrete low pass filter1/Bd(2) ==
  in : Inport
  Constant1 : Constant  Value=variable
  Product1 : Product
  q rounder16 : Subsystem  mask{q=nQ, range=maxRange}
      mask prompts: q "q value"; range "q range"
  out : Outport
  wires:
  q rounder16/1(out) -> Product1/1
  Constant1/1 -> q rounder16/1(in)
  Product1/1 -> out/1
  in/1 -> Product1/2

== system general_charger_2_with_new_rms/control_stage/AC//DC Control/DQ Controller/discrete low pass filter1/Bd(3) ==
  in : Inport
  Constant1 : Constant  Value=variable
  Product1 : Product
  q rounder16 : Subsystem  mask{q=nQ, range=maxRange}
      mask prompts: q "q value"; range "q range"
  out : Outport
  wires:
  q rounder16/1(out) -> Product1/1
  Constant1/1 -> q rounder16/1(in)
  Product1/1 -> out/1
  in/1 -> Product1/2

== system general_charger_2_with_new_rms/control_stage/AC//DC Control/DQ Controller/discrete low pass filter1/Cd(1) ==
  in : Inport
  Constant1 : Constant  Value=variable
  Product1 : Product
  q rounder16 : Subsystem  mask{q=nQ, range=maxRange}
      mask prompts: q "q value"; range "q range"
  out : Outport
  wires:
  q rounder16/1(out) -> Product1/1
  Constant1/1 -> q rounder16/1(in)
  Product1/1 -> out/1
  in/1 -> Product1/2

== system general_charger_2_with_new_rms/control_stage/AC//DC Control/DQ Controller/discrete low pass filter1/Cd(2) ==
  in : Inport
  Constant1 : Constant  Value=variable
  Product1 : Product
  q rounder16 : Subsystem  mask{q=nQ, range=maxRange}
      mask prompts: q "q value"; range "q range"
  out : Outport
  wires:
  q rounder16/1(out) -> Product1/1
  Constant1/1 -> q rounder16/1(in)
  Product1/1 -> out/1
  in/1 -> Product1/2

== system general_charger_2_with_new_rms/control_stage/AC//DC Control/DQ Controller/discrete low pass filter1/Cd(3) ==
  in : Inport
  Constant1 : Constant  Value=variable
  Product1 : Product
  q rounder16 : Subsystem  mask{q=nQ, range=maxRange}
      mask prompts: q "q value"; range "q range"
  out : Outport
  wires:
  q rounder16/1(out) -> Product1/1
  Constant1/1 -> q rounder16/1(in)
  Product1/1 -> out/1
  in/1 -> Product1/2

== system general_charger_2_with_new_rms/control_stage/AC//DC Control/DQ Controller/discrete low pass filter1/Dd ==
  in : Inport
  Constant1 : Constant  Value=variable
  Product1 : Product
  Scope1 : Scope  NumInputPorts=2
      settings: YMin=-5~-5  YMax=5~5
  q rounder16 : Subsystem  mask{q=nQ, range=maxRange}
      mask prompts: q "q value"; range "q range"
  out : Outport
  wires:
  q rounder16/1(out) -> Product1/1, Scope1/2
  Constant1/1 -> Scope1/1, q rounder16/1(in)
  Product1/1 -> out/1
  in/1 -> Product1/2

== system general_charger_2_with_new_rms/control_stage/AC//DC Control/DQ Controller/discrete low pass filter1/q rounder1 ==
  in : Inport
  Gain9 : Gain  Gain=2^-q
  Idealized ADC quantizer : simulink_extras/Additional Discrete/Idealized ADC quantizer  NumberOfConverterBits=32  Vmin=-range  Vmax=range  OutputDataType=double  OutputNegativeValues=on
  out : Outport
  wires:
  in/1 -> Idealized ADC quantizer/1
  Idealized ADC quantizer/1 -> Gain9/1
  Gain9/1 -> out/1

== system general_charger_2_with_new_rms/control_stage/AC//DC Control/DQ Controller/discrete low pass filter1/q rounder10 ==
  in : Inport
  Gain9 : Gain  Gain=2^-q
  Idealized ADC quantizer : simulink_extras/Additional Discrete/Idealized ADC quantizer  NumberOfConverterBits=32  Vmin=-range  Vmax=range  OutputDataType=double  OutputNegativeValues=on
  out : Outport
  wires:
  in/1 -> Idealized ADC quantizer/1
  Idealized ADC quantizer/1 -> Gain9/1
  Gain9/1 -> out/1

== system general_charger_2_with_new_rms/control_stage/AC//DC Control/DQ Controller/discrete low pass filter1/q rounder11 ==
  in : Inport
  Gain9 : Gain  Gain=2^-q
  Idealized ADC quantizer : simulink_extras/Additional Discrete/Idealized ADC quantizer  NumberOfConverterBits=32  Vmin=-range  Vmax=range  OutputDataType=double  OutputNegativeValues=on
  out : Outport
  wires:
  in/1 -> Idealized ADC quantizer/1
  Idealized ADC quantizer/1 -> Gain9/1
  Gain9/1 -> out/1

== system general_charger_2_with_new_rms/control_stage/AC//DC Control/DQ Controller/discrete low pass filter1/q rounder12 ==
  in : Inport
  Gain9 : Gain  Gain=2^-q
  Idealized ADC quantizer : simulink_extras/Additional Discrete/Idealized ADC quantizer  NumberOfConverterBits=32  Vmin=-range  Vmax=range  OutputDataType=double  OutputNegativeValues=on
  out : Outport
  wires:
  in/1 -> Idealized ADC quantizer/1
  Idealized ADC quantizer/1 -> Gain9/1
  Gain9/1 -> out/1

== system general_charger_2_with_new_rms/control_stage/AC//DC Control/DQ Controller/discrete low pass filter1/q rounder13 ==
  in : Inport
  Gain9 : Gain  Gain=2^-q
  Idealized ADC quantizer : simulink_extras/Additional Discrete/Idealized ADC quantizer  NumberOfConverterBits=32  Vmin=-range  Vmax=range  OutputDataType=double  OutputNegativeValues=on
  out : Outport
  wires:
  in/1 -> Idealized ADC quantizer/1
  Idealized ADC quantizer/1 -> Gain9/1
  Gain9/1 -> out/1

== system general_charger_2_with_new_rms/control_stage/AC//DC Control/DQ Controller/discrete low pass filter1/q rounder14 ==
  in : Inport
  Gain9 : Gain  Gain=2^-q
  Idealized ADC quantizer : simulink_extras/Additional Discrete/Idealized ADC quantizer  NumberOfConverterBits=32  Vmin=-range  Vmax=range  OutputDataType=double  OutputNegativeValues=on
  out : Outport
  wires:
  in/1 -> Idealized ADC quantizer/1
  Idealized ADC quantizer/1 -> Gain9/1
  Gain9/1 -> out/1

== system general_charger_2_with_new_rms/control_stage/AC//DC Control/DQ Controller/discrete low pass filter1/q rounder15 ==
  in : Inport
  Gain9 : Gain  Gain=2^-q
  Idealized ADC quantizer : simulink_extras/Additional Discrete/Idealized ADC quantizer  NumberOfConverterBits=32  Vmin=-range  Vmax=range  OutputDataType=double  OutputNegativeValues=on
  out : Outport
  wires:
  in/1 -> Idealized ADC quantizer/1
  Idealized ADC quantizer/1 -> Gain9/1
  Gain9/1 -> out/1

== system general_charger_2_with_new_rms/control_stage/AC//DC Control/DQ Controller/discrete low pass filter1/q rounder16 ==
  in : Inport
  Gain9 : Gain  Gain=2^-q
  Idealized ADC quantizer : simulink_extras/Additional Discrete/Idealized ADC quantizer  NumberOfConverterBits=32  Vmin=-range  Vmax=range  OutputDataType=double  OutputNegativeValues=on
  out : Outport
  wires:
  in/1 -> Idealized ADC quantizer/1
  Idealized ADC quantizer/1 -> Gain9/1
  Gain9/1 -> out/1

== system general_charger_2_with_new_rms/control_stage/AC//DC Control/DQ Controller/discrete low pass filter1/q rounder17 ==
  in : Inport
  Gain9 : Gain  Gain=2^-q
  Idealized ADC quantizer : simulink_extras/Additional Discrete/Idealized ADC quantizer  NumberOfConverterBits=32  Vmin=-range  Vmax=range  OutputDataType=double  OutputNegativeValues=on
  out : Outport
  wires:
  in/1 -> Idealized ADC quantizer/1
  Idealized ADC quantizer/1 -> Gain9/1
  Gain9/1 -> out/1

== system general_charger_2_with_new_rms/control_stage/AC//DC Control/DQ Controller/discrete low pass filter1/q rounder2 ==
  in : Inport
  Gain9 : Gain  Gain=2^-q
  Idealized ADC quantizer : simulink_extras/Additional Discrete/Idealized ADC quantizer  NumberOfConverterBits=32  Vmin=-range  Vmax=range  OutputDataType=double  OutputNegativeValues=on
  out : Outport
  wires:
  in/1 -> Idealized ADC quantizer/1
  Idealized ADC quantizer/1 -> Gain9/1
  Gain9/1 -> out/1

== system general_charger_2_with_new_rms/control_stage/AC//DC Control/DQ Controller/discrete low pass filter1/q rounder3 ==
  in : Inport
  Gain9 : Gain  Gain=2^-q
  Idealized ADC quantizer : simulink_extras/Additional Discrete/Idealized ADC quantizer  NumberOfConverterBits=32  Vmin=-range  Vmax=range  OutputDataType=double  OutputNegativeValues=on
  out : Outport
  wires:
  in/1 -> Idealized ADC quantizer/1
  Idealized ADC quantizer/1 -> Gain9/1
  Gain9/1 -> out/1

== system general_charger_2_with_new_rms/control_stage/AC//DC Control/DQ Controller/discrete low pass filter1/q rounder4 ==
  in : Inport
  Gain9 : Gain  Gain=2^-q
  Idealized ADC quantizer : simulink_extras/Additional Discrete/Idealized ADC quantizer  NumberOfConverterBits=32  Vmin=-range  Vmax=range  OutputDataType=double  OutputNegativeValues=on
  out : Outport
  wires:
  in/1 -> Idealized ADC quantizer/1
  Idealized ADC quantizer/1 -> Gain9/1
  Gain9/1 -> out/1

== system general_charger_2_with_new_rms/control_stage/AC//DC Control/DQ Controller/discrete low pass filter1/q rounder5 ==
  in : Inport
  Gain9 : Gain  Gain=2^-q
  Idealized ADC quantizer : simulink_extras/Additional Discrete/Idealized ADC quantizer  NumberOfConverterBits=32  Vmin=-range  Vmax=range  OutputDataType=double  OutputNegativeValues=on
  out : Outport
  wires:
  in/1 -> Idealized ADC quantizer/1
  Idealized ADC quantizer/1 -> Gain9/1
  Gain9/1 -> out/1

== system general_charger_2_with_new_rms/control_stage/AC//DC Control/DQ Controller/discrete low pass filter1/q rounder6 ==
  in : Inport
  Gain9 : Gain  Gain=2^-q
  Idealized ADC quantizer : simulink_extras/Additional Discrete/Idealized ADC quantizer  NumberOfConverterBits=32  Vmin=-range  Vmax=range  OutputDataType=double  OutputNegativeValues=on
  out : Outport
  wires:
  in/1 -> Idealized ADC quantizer/1
  Idealized ADC quantizer/1 -> Gain9/1
  Gain9/1 -> out/1

== system general_charger_2_with_new_rms/control_stage/AC//DC Control/DQ Controller/discrete low pass filter1/q rounder7 ==
  in : Inport
  Gain9 : Gain  Gain=2^-q
  Idealized ADC quantizer : simulink_extras/Additional Discrete/Idealized ADC quantizer  NumberOfConverterBits=32  Vmin=-range  Vmax=range  OutputDataType=double  OutputNegativeValues=on
  out : Outport
  wires:
  in/1 -> Idealized ADC quantizer/1
  Idealized ADC quantizer/1 -> Gain9/1
  Gain9/1 -> out/1

== system general_charger_2_with_new_rms/control_stage/AC//DC Control/DQ Controller/discrete low pass filter1/q rounder8 ==
  in : Inport
  Gain9 : Gain  Gain=2^-q
  Idealized ADC quantizer : simulink_extras/Additional Discrete/Idealized ADC quantizer  NumberOfConverterBits=32  Vmin=-range  Vmax=range  OutputDataType=double  OutputNegativeValues=on
  out : Outport
  wires:
  in/1 -> Idealized ADC quantizer/1
  Idealized ADC quantizer/1 -> Gain9/1
  Gain9/1 -> out/1

== system general_charger_2_with_new_rms/control_stage/AC//DC Control/DQ Controller/discrete low pass filter1/q rounder9 ==
  in : Inport
  Gain9 : Gain  Gain=2^-q
  Idealized ADC quantizer : simulink_extras/Additional Discrete/Idealized ADC quantizer  NumberOfConverterBits=32  Vmin=-range  Vmax=range  OutputDataType=double  OutputNegativeValues=on
  out : Outport
  wires:
  in/1 -> Idealized ADC quantizer/1
  Idealized ADC quantizer/1 -> Gain9/1
  Gain9/1 -> out/1

== system general_charger_2_with_new_rms/control_stage/AC//DC Control/PR Controller/Source Voltage PLL/AB->DQ ==
  A : Inport
  wt : Inport  Port=2
  Add1 : Sum  Inputs=-+
  Add2 : Sum
  Delay : Delay  DelayLength=round(1/f/4/Ts)  SampleTime=Ts
  Product{1..4} (4 alike) : Product  RndMeth=Zero
  Trigonometric Function : Trigonometry
  Trigonometric Function1 : Trigonometry  Operator=cos
  D : Outport
  Q : Outport  Port=2
  wires:
  Add2/1 -> D/1  "Vd"
  Trigonometric Function/1 -> Product2/1, Product1/1
  Product1/1 -> Add2/2
  Product4/1 -> Add2/1
  wt/1 -> Trigonometric Function1/1, Trigonometric Function/1
  Delay/1 -> Product1/2, Product3/2
  Product2/1 -> Add1/1
  Product3/1 -> Add1/2
  Add1/1 -> Q/1
  A/1 -> Delay/1, Product4/1, Product2/2
  Trigonometric Function1/1 -> Product3/1, Product4/2

== system general_charger_2_with_new_rms/control_stage/AC//DC Control/PR Controller/Source Voltage PLL/PI2 ==
  in : Inport
  Add1 : Sum
  Add2 : Sum
  Ki : Gain  Gain=ki
  Kp : Gain  Gain=kp
  Tappe : simulink/Discrete/Tapped Delay  vinit=0.0  samptime=Ts_pi  NumDelays=1  DelayOrder=Oldest  includeCurrent=off
  Ts : Gain  Gain=Ts_pi
  integral saturation : Saturate  UpperLimit=int_sat_up  LowerLimit=int_sat_low  SampleTime=Ts_pi
  pi controller saturation : Saturate  UpperLimit=pi_sat_up  LowerLimit=pi_sat_low  SampleTime=Ts_pi
  out : Outport
  wires:
  Ts/1 -> Ki/1
  in/1 -> Kp/1, Ts/1  "vdc_error"
  Add1/1 -> integral saturation/1  "vdc_int_pi"
  Kp/1 -> Add2/2  "vdc_kp_pi"
  pi controller saturation/1 -> out/1
  Tappe/1 -> Add1/1
  Add2/1 -> pi controller saturation/1  "vdc_pi"
  Ki/1 -> Add1/2
  integral saturation/1 -> Add2/1, Tappe/1

== system general_charger_2_with_new_rms/Measurements/Power and angle calculations/AB-DQ Transform/Vab_dq/AB->DQ/Vd Discretization Error Correction ==
  A : Inport
  wt : Inport  Port=2
  D : Inport  Port=3
  Add1 : Sum  Inputs=-+
  Add2 : Sum  Inputs=-+
  Gain2 : Gain  Gain=0.000078956
  Gain3 : Gain  Gain=0.012566039
  Product : Product
  Product1 : Product
  Product2 : Product
  Trigonometric Function : Trigonometry
  Trigonometric Function1 : Trigonometry
  Trigonometric Function2 : Trigonometry
  Trigonometric Function3 : Trigonometry  Operator=cos
  Vd_corr : Outport
  wires:
  Add1/1 -> Product2/2
  Add2/1 -> Vd_corr/1
  A/1 -> Product2/1
  wt/1 -> Trigonometric Function2/1, Trigonometric Function3/1, Trigonometric Function/1, Trigonometric Function1/1
  Trigonometric Function/1 -> Product/2
  Trigonometric Function3/1 -> Product1/2
  Product1/1 -> Gain3/1
  Product2/1 -> Add2/1
  Trigonometric Function1/1 -> Product/1
  Product/1 -> Gain2/1
  D/1 -> Add2/2
  Gain3/1 -> Add1/1
  Trigonometric Function2/1 -> Product1/1
  Gain2/1 -> Add1/2
